simulink library "foc_blocks"  (R2020b)
settings: Solver=ode45  StartTime=0.0  StopTime=10.0  RelTol=1e-3  EnableMultiTasking=on
values from neighbouring files (symbols this model uses):
  ClockFrequency = 100    [setup_DF_fixp16_alu_av.m]    (also in setup_sim_DF_fixp16_alu.m; setup_verify_DF_fixp16_alu.m)
  constfractionlengthIn = 10    [setup_DF_fixp16_alu_av.m]    (also in setup_sim_DF_fixp16_alu.m; setup_verify_DF_fixp16_alu.m)
  constwordlengthIn = 16    [setup_DF_fixp16_alu_av.m]    (also in setup_sim_DF_fixp16_alu.m; setup_verify_DF_fixp16_alu.m)
  DSPBASampleTime = FoldingFactor / (ClockFrequency * 1e6)    (= 5e-06)    [setup_DF_fixp16_alu_av.m]    (also in setup_sim_DF_fixp16_alu.m; setup_verify_DF_fixp16_alu.m)
  FoldingFactor = 500    [setup_DF_fixp16_alu_av.m]    (also in setup_sim_DF_fixp16_alu.m; setup_verify_DF_fixp16_alu.m)
undefined symbols (not defined in the file or in its folder): AdvDSPBChannelOutDisplay, dpoly, dspba_ChannelInVis, dspba_ChannelOutVis, dspba_internal_get_channel_ports, evalAionMaskParam, latency, primtype, value, x
libraries: DSPBAPrim x559, AlteraGenericMotorLibrary x20, $bdroot x9, DSPBAUtilities x4, DSPBAControl x4
(part 3 of 6)

== system foc_blocks/FL_fixp16/SVM ==
  tmax : Inport
  ABin : Inport  Port=2
  Convert1 : DSPBAPrim/Convert  primtype=convert  nInputs=1  nOutputs=1  omode=Specify via dialog  otype=sfix(32)  scale=2^-0  rndmethod=Biased  factor=1  satmethod=None  shift_vec=[0 1 2 -1]  value=round([0:255]/17)  inPortNames=[' '; ' ';]  outPortNames=[' '; 'c']  dspbaimage=dspba_prim.jpg  text=fprintf('convert');  style=Optimised  visibilities=8+64+256+2^17  clipdetect=off  floatPrecision=float32_m23  advOptions=[]  version=20130211
  Demux : Demux  Outputs=2
  Mod : Subsystem
  Mult : DSPBAPrim/Mult  primtype=mult  nInputs=2  nOutputs=1  omode=Inherit via internal rule  otype=constOTypeMult  scale=constScaleIn  rndmethod=Unbiased  factor=1  satmethod=Symmetric  shift_vec=[0 1 2 -1]  value=0  inPortNames=[' '; ' ';]  outPortNames=[' ']  dspbaimage=dspba_prim.jpg  text=fprintf('X');  style=Optimised  visibilities=8  floatPrecision=float32_m23  floatRounding=correct  advOptions=[]  version=20130115
  Mux : Mux  Inputs=3
  ReinterpretCast1 : DSPBAPrim/ReinterpretCast  primtype=reinterpret  nInputs=1  nOutputs=1  omode=Specify via dialog  otype=sfix(33)  scale=2^-15  rndmethod=Unbiased  factor=1  satmethod=Symmetric  shift_vec=[0 1 2 -1]  value=0  inPortNames=[' '; ' ';]  outPortNames=[' ']  dspbaimage=dspba_prim.jpg  text=fprintf('Reinterp\nCast', value);  style=Optimised  visibilities=8  floatPrecision=float32_m23  version=20120601
  SectorSel : Subsystem
  rotv : Subsystem
  Out_uvw : Outport
  Out_sect : Outport  Port=2
  wires:
  Convert1/1 -> Demux/1
  ReinterpretCast1/1 -> Convert1/1
  Mult/1 -> ReinterpretCast1/1
  Mod/3(Out_w) -> Mux/3
  Mod/2(Out_v) -> Mux/2
  tmax/1 -> Mod/5(Max), Mult/2
  Mod/1(Out_u) -> Mux/1
  rotv/5(D3BA) -> Mod/8(B3m)
  rotv/6(S3BAm) -> Mod/7(B3p)
  rotv/4(uA) -> Mod/6(A)
  Demux/2 -> rotv/2(Bin), SectorSel/2(B)
  rotv/1(S) -> SectorSel/3(Sum), Mod/4(Sum)
  rotv/3(uB) -> Mod/2(B)
  rotv/2(DBA) -> SectorSel/1(D), Mod/1(D)
  Demux/1 -> rotv/1(Ain)
  ABin/1 -> Mult/1
  Mux/1 -> Out_uvw/1
  SectorSel/1(sel) -> Mod/3(Sel), Out_sect/1

== system foc_blocks/FL_fixp16_filt/FP_CP1_DSPBA ==
  note: Park & Clarke Transform
  note: Feedback Current
  note: Sin/Cos Electrical Angle
  I_uw : Inport
  cos_phi_el : Inport  Port=2
  sin_phi_el : Inport  Port=3
  Add : DSPBAPrim/Add  primtype=add  nInputs=evalAionMaskParam(gcb,'value',1)  nOutputs=1  omode=Inherit via internal rule  otype=sfix(16)  scale=2^-15  rndmethod=Unbiased  factor=1  satmethod=Symmetric  shift_vec=[0 1 2 -1]  value=2  inPortNames=[' '; ' ';]  outPortNames=[' ']  dspbaimage=dspba_prim.jpg  text=fprintf('+');  style=Optimised  visibilities=1032  genFPC=off  floatRounding=correct  advOptions=[]  version=20130821
  Add1 : DSPBAPrim/Add  primtype=add  nInputs=evalAionMaskParam(gcb,'value',1)  nOutputs=1  omode=Inherit via internal rule  otype=sfix(16)  scale=2^-15  rndmethod=Unbiased  factor=1  satmethod=Symmetric  shift_vec=[0 1 2 -1]  value=2  inPortNames=[' '; ' ';]  outPortNames=[' ']  dspbaimage=dspba_prim.jpg  text=fprintf('+');  style=Optimised  visibilities=1032  genFPC=off  floatRounding=correct  advOptions=[]  version=20130821
  Altera DSP Builder Advanced : AlteraGenericMotorLibrary/FP_Cur_Ctrl_DSPBA/Altera DSP Builder Advanced  SystemSampleTime=-1  VariantActivationTime=update diagram  Latency=0  AutoFrameSizeCalculation=off
  Demux1 : Demux  Outputs=2
  FixedGain : Subsystem  mask{constVal=2}
      mask prompts: constVal "Gain"
      mask Display: color('w');fprintf('Fixed Gain\n%s', num2str(constVal));port_label('input',1,'a');port_label('output',1,'q');
  FixedGain1 : Subsystem  mask{constVal=-1/sqrt(3)}
      mask prompts: constVal "Gain"
      mask Display: color('w');fprintf('Fixed Gain\n%s', num2str(constVal));port_label('input',1,'a');port_label('output',1,'q');
  Mult{,1..3} (4 alike) : DSPBAPrim/Mult  primtype=mult  nInputs=2  nOutputs=1  omode=Specify via dialog  otype=constOTypeIn  scale=constScaleIn  rndmethod=Unbiased  factor=1  satmethod=Symmetric  shift_vec=[0 1 2 -1]  value=0  inPortNames=[' '; ' ';]  outPortNames=[' ']  dspbaimage=dspba_prim.jpg  text=fprintf('X');  style=Optimised  visibilities=8  floatPrecision=float32_m23  floatRounding=correct  advOptions=[]  version=20130115
  Mux1 : Mux  Inputs=2
  Sub1 : DSPBAPrim/Sub  primtype=sub  nInputs=2  nOutputs=1  omode=Inherit via internal rule  otype=sfix(16)  scale=2^-15  rndmethod=Unbiased  factor=1  satmethod=Symmetric  shift_vec=[0 1 2 -1]  value=0  inPortNames=['+'; '-';]  outPortNames=[' ']  dspbaimage=dspba_prim.jpg  text=fprintf('-');  style=Optimised  visibilities=8  floatRounding=correct  advOptions=[]  version=20130115
  I_dq : Outport
  wires:
  Sub1/1 -> Mux1/2
  Add/1 -> Mux1/1
  Mux1/1 -> I_dq/1
  Mult3/1 -> Sub1/1
  Mult2/1 -> Sub1/2
  Mult1/1 -> Add/2
  Mult/1 -> Add/1
  cos_phi_el/1 -> Mult/2, Mult3/2
  FixedGain1/1(Out1) -> Mult1/1, Mult3/1
  Demux1/1 -> Mult/1, Mult2/2, Add1/1
  Demux1/2 -> FixedGain/1(In1)
  I_uw/1 -> Demux1/1
  sin_phi_el/1 -> Mult1/2, Mult2/1
  Add1/1 -> FixedGain1/1(In1)
  FixedGain/1(Out1) -> Add1/2

== system foc_blocks/FL_fixp16_filt/FP_Inv_Park ==
  note: Inverse Park Transform
  note: Sin/Cos Electrical Angle
  note: Direct/Quadrature Voltage
  note: Alpha/Beta Voltage
  V_dq : Inport
  cos_phi_el : Inport  Port=2
  sin_phi_el : Inport  Port=3
  Add : DSPBAPrim/Add  primtype=add  nInputs=evalAionMaskParam(gcb,'value',1)  nOutputs=1  omode=Inherit via internal rule with word growth  otype=sfix(16)  scale=2^-15  rndmethod=Unbiased  factor=1  satmethod=Symmetric  shift_vec=[0 1 2 -1]  value=2  inPortNames=[' '; ' ';]  outPortNames=[' ']  dspbaimage=dspba_prim.jpg  text=fprintf('+');  style=Optimised  visibilities=1032  genFPC=off  floatRounding=correct  advOptions=[]  version=20130821
  Altera DSP Builder Advanced : AlteraGenericMotorLibrary/FP_Cur_Ctrl_DSPBA/Altera DSP Builder Advanced  SystemSampleTime=-1  VariantActivationTime=update diagram  Latency=0  AutoFrameSizeCalculation=off
  Demux1 : Demux  Outputs=2
  Mult{,1..3} (4 alike) : DSPBAPrim/Mult  primtype=mult  nInputs=2  nOutputs=1  omode=Specify via dialog  otype=constOTypeMult  scale=constScaleIn  rndmethod=Unbiased  factor=1  satmethod=Symmetric  shift_vec=[0 1 2 -1]  value=0  inPortNames=[' '; ' ';]  outPortNames=[' ']  dspbaimage=dspba_prim.jpg  text=fprintf('X');  style=Optimised  visibilities=8  floatPrecision=float32_m23  floatRounding=correct  advOptions=[]  version=20130115
  Mux2 : Mux  Inputs=2
  Sub1 : DSPBAPrim/Sub  primtype=sub  nInputs=2  nOutputs=1  omode=Inherit via internal rule with word growth  otype=sfix(16)  scale=2^-15  rndmethod=Unbiased  factor=1  satmethod=Symmetric  shift_vec=[0 1 2 -1]  value=0  inPortNames=['+'; '-';]  outPortNames=[' ']  dspbaimage=dspba_prim.jpg  text=fprintf('-');  style=Optimised  visibilities=8  floatRounding=correct  advOptions=[]  version=20130115
  V_alpha_beta : Outport
  wires:
  Mult2/1 -> Add/1
  Mult3/1 -> Add/2
  Mult/1 -> Sub1/1
  Mult1/1 -> Sub1/2
  Demux1/1 -> Mult/1, Mult2/1  "I_d"
  cos_phi_el/1 -> Mult/2, Mult3/2
  Demux1/2 -> Mult1/1, Mult3/1  "I_q"
  sin_phi_el/1 -> Mult1/2, Mult2/2
  V_dq/1 -> Demux1/1
  Mux2/1 -> V_alpha_beta/1
  Sub1/1 -> Mux2/1
  Add/1 -> Mux2/2

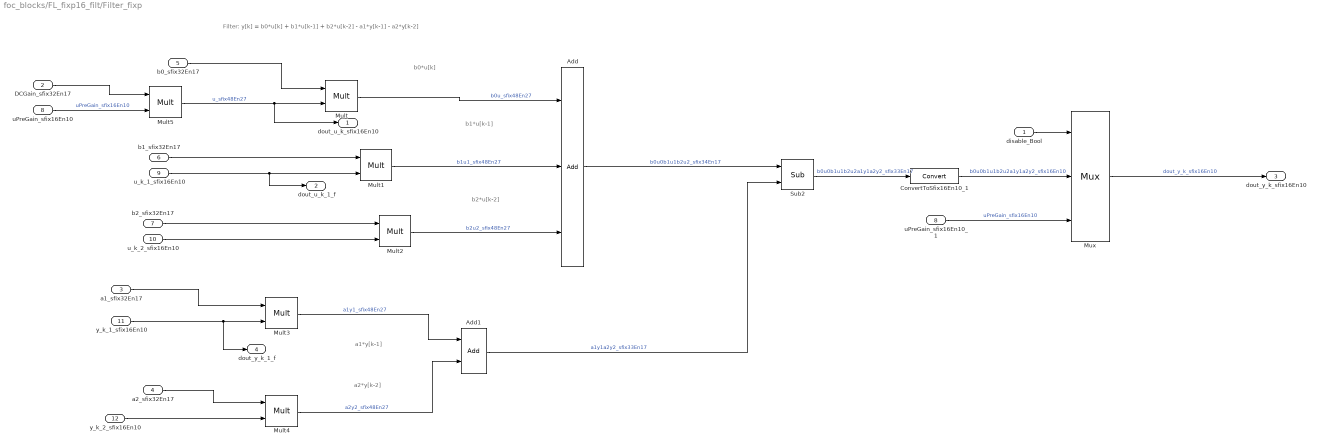
== system foc_blocks/FL_fixp16_filt/Filter_fixp ==
  note: b0*u[k]
  note: b1*u[k-1]
  note: b2*u[k-2]
  note: a1*y[k-1]
  note: a2*y[k-2]
  note: Filter: y[k] = b0*u[k] + b1*u[k-1] + b2*u[k-2] - a1*y[k-1] - a2*y[k-2]
  disable_Bool : Inport
  DCGain_sfix32En17 : Inport  Port=2
  a1_sfix32En17 : Inport  Port=3
  a2_sfix32En17 : Inport  Port=4
  b0_sfix32En17 : Inport  Port=5
  b1_sfix32En17 : Inport  Port=6
  b2_sfix32En17 : Inport  Port=7
  uPreGain_sfix16En10 : Inport  Port=8
  u_k_1_sfix16En10 : Inport  Port=9
  u_k_2_sfix16En10 : Inport  Port=10
  y_k_1_sfix16En10 : Inport  Port=11
  y_k_2_sfix16En10 : Inport  Port=12
  Add : DSPBAPrim/Add  primtype=add  nInputs=evalAionMaskParam(gcb,'value',1)  nOutputs=1  omode=Inherit via internal rule  otype=sfix(16)  scale=2^-15  rndmethod=Unbiased  factor=1  satmethod=Symmetric  shift_vec=[0 1 2 -1]  value=3  inPortNames=[' '; ' ';]  outPortNames=[' ']  dspbaimage=dspba_prim.jpg  text=fprintf('+');  style=Optimised  visibilities=1032  genFPC=off  floatRounding=correct  advOptions=[]  version=20130821
  Add1 : DSPBAPrim/Add  primtype=add  nInputs=evalAionMaskParam(gcb,'value',1)  nOutputs=1  omode=Inherit via internal rule  otype=sfix(16)  scale=2^-15  rndmethod=Unbiased  factor=1  satmethod=Symmetric  shift_vec=[0 1 2 -1]  value=2  inPortNames=[' '; ' ';]  outPortNames=[' ']  dspbaimage=dspba_prim.jpg  text=fprintf('+');  style=Optimised  visibilities=1032  genFPC=off  floatRounding=correct  advOptions=[]  version=20130821
  ConvertToSfix16En10_1 : DSPBAPrim/Convert  primtype=convert  nInputs=1  nOutputs=1  omode=Specify via dialog  otype=constOTypeIn  scale=constScaleIn  rndmethod=Truncate  factor=1  satmethod=None  shift_vec=[0 1 2 -1]  value=round([0:255]/17)  inPortNames=[' '; ' ';]  outPortNames=[' '; 'c']  dspbaimage=dspba_prim.jpg  text=fprintf('convert');  style=Optimised  visibilities=8+64+256+2^17  clipdetect=off  floatPrecision=float32_m23  advOptions=[]  version=20130211
  Mult{,1..4} (5 alike) : DSPBAPrim/Mult  primtype=mult  nInputs=2  nOutputs=1  omode=Specify via dialog  otype=constOTypeFilterCoeffs  scale=constScaleFilterCoeffs  rndmethod=Unbiased  factor=1  satmethod=Symmetric  shift_vec=[0 1 2 -1]  value=0  inPortNames=[' '; ' ';]  outPortNames=[' ']  dspbaimage=dspba_prim.jpg  text=fprintf('X');  style=Optimised  visibilities=8  floatPrecision=float32_m23  floatRounding=correct  advOptions=[]  version=20130115
  Mult5 : DSPBAPrim/Mult  primtype=mult  nInputs=2  nOutputs=1  omode=Specify via dialog  otype=constOTypeIn  scale=constScaleIn  rndmethod=Unbiased  factor=1  satmethod=Symmetric  shift_vec=[0 1 2 -1]  value=0  inPortNames=[' '; ' ';]  outPortNames=[' ']  dspbaimage=dspba_prim.jpg  text=fprintf('X');  style=Optimised  visibilities=8  floatPrecision=float32_m23  floatRounding=correct  advOptions=[]  version=20130115
  Mux : DSPBAPrim/Mux  primtype=mux  nInputs=evalAionMaskParam(gcb,'value',1)+1  nOutputs=1  omode=Inherit via internal rule  otype=constOTypeFromFOC  scale=constScaleFromFOC  rndmethod=Unbiased  factor=1  satmethod=Symmetric  shift_vec=[0 1 2 -1]  value=2  inPortNames=['s'; 'd0'; 'd1'; 'd2'; 'd3'; 'd4'; 'd5'; 'd6'; 'd7'; 'd8'; 'd9';]  outPortNames=[' ']  dspbaimage=dspba_prim.jpg  text=fprintf('%s', primtype);  style=Optimised  visibilities=1032  version=20131025
  Sub2 : DSPBAPrim/Sub  primtype=sub  nInputs=2  nOutputs=1  omode=Inherit via internal rule  otype=sfix(16)  scale=2^-15  rndmethod=Unbiased  factor=1  satmethod=Symmetric  shift_vec=[0 1 2 -1]  value=0  inPortNames=['+'; '-';]  outPortNames=[' ']  dspbaimage=dspba_prim.jpg  text=fprintf('-');  style=Optimised  visibilities=8  floatRounding=correct  advOptions=[]  version=20130115
  uPreGain_sfix16En10_1 : InportShadow  Port=8
  dout_u_k_sfix16En10 : Outport
  dout_u_k_1_f : Outport  Port=2
  dout_y_k_sfix16En10 : Outport  Port=3
  dout_y_k_1_f : Outport  Port=4
  wires:
  Mult4/1 -> Add1/2  "a2y2_sfix48En27"
  Mult3/1 -> Add1/1  "a1y1_sfix48En27"
  Add1/1 -> Sub2/2  "a1y1a2y2_sfix33En17"
  Add/1 -> Sub2/1  "b0u0b1u1b2u2_sfix34En17"
  Mult1/1 -> Add/2  "b1u1_sfix48En27"
  Mult/1 -> Add/1  "b0u_sfix48En27"
  Mult2/1 -> Add/3  "b2u2_sfix48En27"
  Mult5/1 -> dout_u_k_sfix16En10/1, Mult/2  "u_sfix48En27"
  disable_Bool/1 -> Mux/1
  Sub2/1 -> ConvertToSfix16En10_1/1  "b0u0b1u1b2u2a1y1a2y2_sfix33En17"
  Mux/1 -> dout_y_k_sfix16En10/1  "dout_y_k_sfix16En10"
  DCGain_sfix32En17/1 -> Mult5/1
  uPreGain_sfix16En10/1 -> Mult5/2  "uPreGain_sfix16En10"
  uPreGain_sfix16En10_1/1 -> Mux/3  "uPreGain_sfix16En10"
  b0_sfix32En17/1 -> Mult/1
  b2_sfix32En17/1 -> Mult2/1
  b1_sfix32En17/1 -> Mult1/1
  a1_sfix32En17/1 -> Mult3/1
  a2_sfix32En17/1 -> Mult4/1
  ConvertToSfix16En10_1/1 -> Mux/2  "b0u0b1u1b2u2a1y1a2y2_sfix16En10"
  u_k_1_sfix16En10/1 -> dout_u_k_1_f/1, Mult1/2
  u_k_2_sfix16En10/1 -> Mult2/2
  y_k_1_sfix16En10/1 -> dout_y_k_1_f/1, Mult3/2
  y_k_2_sfix16En10/1 -> Mult4/2

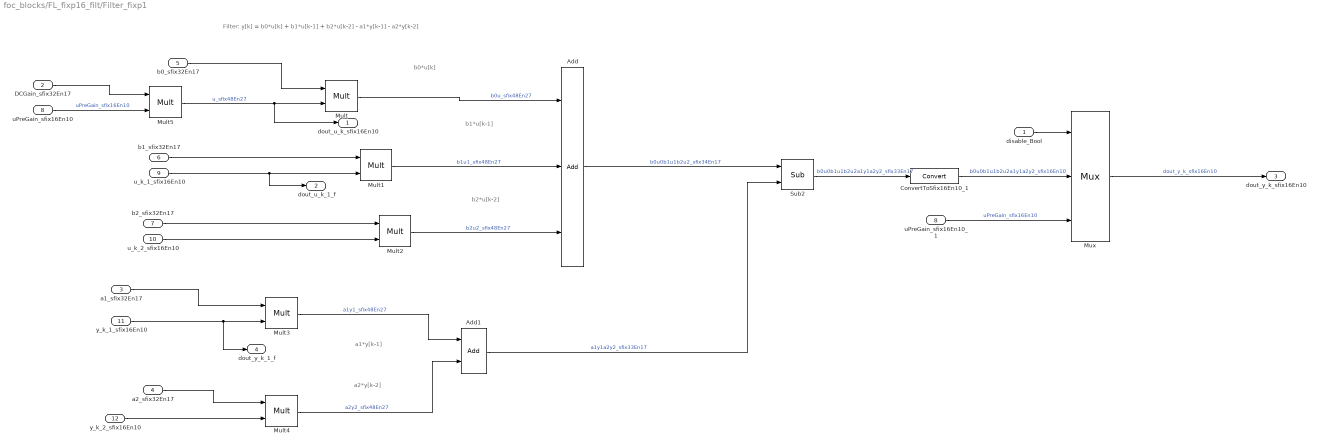
== system foc_blocks/FL_fixp16_filt/Filter_fixp1 ==
  note: b0*u[k]
  note: b1*u[k-1]
  note: b2*u[k-2]
  note: a1*y[k-1]
  note: a2*y[k-2]
  note: Filter: y[k] = b0*u[k] + b1*u[k-1] + b2*u[k-2] - a1*y[k-1] - a2*y[k-2]
  disable_Bool : Inport
  DCGain_sfix32En17 : Inport  Port=2
  a1_sfix32En17 : Inport  Port=3
  a2_sfix32En17 : Inport  Port=4
  b0_sfix32En17 : Inport  Port=5
  b1_sfix32En17 : Inport  Port=6
  b2_sfix32En17 : Inport  Port=7
  uPreGain_sfix16En10 : Inport  Port=8
  u_k_1_sfix16En10 : Inport  Port=9
  u_k_2_sfix16En10 : Inport  Port=10
  y_k_1_sfix16En10 : Inport  Port=11
  y_k_2_sfix16En10 : Inport  Port=12
  Add : DSPBAPrim/Add  primtype=add  nInputs=evalAionMaskParam(gcb,'value',1)  nOutputs=1  omode=Inherit via internal rule  otype=sfix(16)  scale=2^-15  rndmethod=Unbiased  factor=1  satmethod=Symmetric  shift_vec=[0 1 2 -1]  value=3  inPortNames=[' '; ' ';]  outPortNames=[' ']  dspbaimage=dspba_prim.jpg  text=fprintf('+');  style=Optimised  visibilities=1032  genFPC=off  floatRounding=correct  advOptions=[]  version=20130821
  Add1 : DSPBAPrim/Add  primtype=add  nInputs=evalAionMaskParam(gcb,'value',1)  nOutputs=1  omode=Inherit via internal rule  otype=sfix(16)  scale=2^-15  rndmethod=Unbiased  factor=1  satmethod=Symmetric  shift_vec=[0 1 2 -1]  value=2  inPortNames=[' '; ' ';]  outPortNames=[' ']  dspbaimage=dspba_prim.jpg  text=fprintf('+');  style=Optimised  visibilities=1032  genFPC=off  floatRounding=correct  advOptions=[]  version=20130821
  ConvertToSfix16En10_1 : DSPBAPrim/Convert  primtype=convert  nInputs=1  nOutputs=1  omode=Specify via dialog  otype=constOTypeIn  scale=constScaleIn  rndmethod=Truncate  factor=1  satmethod=None  shift_vec=[0 1 2 -1]  value=round([0:255]/17)  inPortNames=[' '; ' ';]  outPortNames=[' '; 'c']  dspbaimage=dspba_prim.jpg  text=fprintf('convert');  style=Optimised  visibilities=8+64+256+2^17  clipdetect=off  floatPrecision=float32_m23  advOptions=[]  version=20130211
  Mult{,1..4} (5 alike) : DSPBAPrim/Mult  primtype=mult  nInputs=2  nOutputs=1  omode=Specify via dialog  otype=constOTypeFilterCoeffs  scale=constScaleFilterCoeffs  rndmethod=Unbiased  factor=1  satmethod=Symmetric  shift_vec=[0 1 2 -1]  value=0  inPortNames=[' '; ' ';]  outPortNames=[' ']  dspbaimage=dspba_prim.jpg  text=fprintf('X');  style=Optimised  visibilities=8  floatPrecision=float32_m23  floatRounding=correct  advOptions=[]  version=20130115
  Mult5 : DSPBAPrim/Mult  primtype=mult  nInputs=2  nOutputs=1  omode=Specify via dialog  otype=constOTypeIn  scale=constScaleIn  rndmethod=Unbiased  factor=1  satmethod=Symmetric  shift_vec=[0 1 2 -1]  value=0  inPortNames=[' '; ' ';]  outPortNames=[' ']  dspbaimage=dspba_prim.jpg  text=fprintf('X');  style=Optimised  visibilities=8  floatPrecision=float32_m23  floatRounding=correct  advOptions=[]  version=20130115
  Mux : DSPBAPrim/Mux  primtype=mux  nInputs=evalAionMaskParam(gcb,'value',1)+1  nOutputs=1  omode=Inherit via internal rule  otype=constOTypeFromFOC  scale=constScaleFromFOC  rndmethod=Unbiased  factor=1  satmethod=Symmetric  shift_vec=[0 1 2 -1]  value=2  inPortNames=['s'; 'd0'; 'd1'; 'd2'; 'd3'; 'd4'; 'd5'; 'd6'; 'd7'; 'd8'; 'd9';]  outPortNames=[' ']  dspbaimage=dspba_prim.jpg  text=fprintf('%s', primtype);  style=Optimised  visibilities=1032  version=20131025
  Sub2 : DSPBAPrim/Sub  primtype=sub  nInputs=2  nOutputs=1  omode=Inherit via internal rule  otype=sfix(16)  scale=2^-15  rndmethod=Unbiased  factor=1  satmethod=Symmetric  shift_vec=[0 1 2 -1]  value=0  inPortNames=['+'; '-';]  outPortNames=[' ']  dspbaimage=dspba_prim.jpg  text=fprintf('-');  style=Optimised  visibilities=8  floatRounding=correct  advOptions=[]  version=20130115
  uPreGain_sfix16En10_1 : InportShadow  Port=8
  dout_u_k_sfix16En10 : Outport
  dout_u_k_1_f : Outport  Port=2
  dout_y_k_sfix16En10 : Outport  Port=3
  dout_y_k_1_f : Outport  Port=4
  wires:
  Mult4/1 -> Add1/2  "a2y2_sfix48En27"
  Mult3/1 -> Add1/1  "a1y1_sfix48En27"
  Add1/1 -> Sub2/2  "a1y1a2y2_sfix33En17"
  Add/1 -> Sub2/1  "b0u0b1u1b2u2_sfix34En17"
  Mult1/1 -> Add/2  "b1u1_sfix48En27"
  Mult/1 -> Add/1  "b0u_sfix48En27"
  Mult2/1 -> Add/3  "b2u2_sfix48En27"
  Mult5/1 -> dout_u_k_sfix16En10/1, Mult/2  "u_sfix48En27"
  disable_Bool/1 -> Mux/1
  Sub2/1 -> ConvertToSfix16En10_1/1  "b0u0b1u1b2u2a1y1a2y2_sfix33En17"
  Mux/1 -> dout_y_k_sfix16En10/1  "dout_y_k_sfix16En10"
  DCGain_sfix32En17/1 -> Mult5/1
  uPreGain_sfix16En10/1 -> Mult5/2  "uPreGain_sfix16En10"
  uPreGain_sfix16En10_1/1 -> Mux/3  "uPreGain_sfix16En10"
  b0_sfix32En17/1 -> Mult/1
  b2_sfix32En17/1 -> Mult2/1
  b1_sfix32En17/1 -> Mult1/1
  a1_sfix32En17/1 -> Mult3/1
  a2_sfix32En17/1 -> Mult4/1
  ConvertToSfix16En10_1/1 -> Mux/2  "b0u0b1u1b2u2a1y1a2y2_sfix16En10"
  u_k_1_sfix16En10/1 -> dout_u_k_1_f/1, Mult1/2
  u_k_2_sfix16En10/1 -> Mult2/2
  y_k_1_sfix16En10/1 -> dout_y_k_1_f/1, Mult3/2
  y_k_2_sfix16En10/1 -> Mult4/2

== system foc_blocks/FL_fixp16_filt/Fixed Saturate1 ==
  In1 : Inport
  limit : Inport  Port=2
  MinMax : DSPBAPrim/MinMax  primtype=minmaxfunc  nInputs=2  nOutputs=1  omode=Specify via dialog  otype=constOTypeIn  scale=constScaleIn  rndmethod=Unbiased  factor=1  satmethod=Symmetric  shift_vec=[0 1 2 -1]  value=0  inPortNames=[' '; ' ';]  outPortNames=[' ']  dspbaimage=dspba_prim.jpg  text=disp('min');  style=Optimised  visibilities=8+2^17  functionExpr=min  advOptions=[]  version=20121130
  MinMax1 : DSPBAPrim/MinMax  primtype=minmaxfunc  nInputs=2  nOutputs=1  omode=Specify via dialog  otype=constOTypeIn  scale=constScaleIn  rndmethod=Unbiased  factor=1  satmethod=Symmetric  shift_vec=[0 1 2 -1]  value=0  inPortNames=[' '; ' ';]  outPortNames=[' ']  dspbaimage=dspba_prim.jpg  text=disp('min');  style=Optimised  visibilities=8+2^17  functionExpr=max  advOptions=[]  version=20121130
  Sub : DSPBAPrim/Sub  primtype=sub  nInputs=2  nOutputs=1  omode=Inherit via internal rule  otype=sfix(16)  scale=2^-15  rndmethod=Unbiased  factor=1  satmethod=Symmetric  shift_vec=[0 1 2 -1]  value=0  inPortNames=['+'; '-';]  outPortNames=[' ']  dspbaimage=dspba_prim.jpg  text=fprintf('-');  style=Optimised  visibilities=8  floatRounding=correct  advOptions=[]  version=20130115
  const1 : DSPBAPrim/Const  primtype=const  nInputs=0  nOutputs=1  omode=Specify via dialog  otype=constOTypeIn  scale=constScaleIn  rndmethod=Unbiased  factor=1  satmethod=Symmetric  shift_vec=[0 1 2 -1]  value=0  inPortNames=['+'; '+';]  outPortNames=[' ']  dspbaimage=dspba_prim.jpg  text=fprintf('%s', num2str(value));  style=Optimised  visibilities=8 + 1024  floatPrecision=float32_m23  version=20120820
  Out1 : Outport
  wires:
  limit/1 -> MinMax/1, Sub/2
  const1/1 -> Sub/1
  In1/1 -> MinMax/2
  Sub/1 -> MinMax1/2
  MinMax1/1 -> Out1/1
  MinMax/1 -> MinMax1/1

== system foc_blocks/FL_fixp16_filt/Fixed Saturate2 ==
  In1 : Inport
  limit : Inport  Port=2
  MinMax : DSPBAPrim/MinMax  primtype=minmaxfunc  nInputs=2  nOutputs=1  omode=Specify via dialog  otype=constOTypeIn  scale=constScaleIn  rndmethod=Unbiased  factor=1  satmethod=Symmetric  shift_vec=[0 1 2 -1]  value=0  inPortNames=[' '; ' ';]  outPortNames=[' ']  dspbaimage=dspba_prim.jpg  text=disp('min');  style=Optimised  visibilities=8+2^17  functionExpr=min  advOptions=[]  version=20121130
  MinMax1 : DSPBAPrim/MinMax  primtype=minmaxfunc  nInputs=2  nOutputs=1  omode=Specify via dialog  otype=constOTypeIn  scale=constScaleIn  rndmethod=Unbiased  factor=1  satmethod=Symmetric  shift_vec=[0 1 2 -1]  value=0  inPortNames=[' '; ' ';]  outPortNames=[' ']  dspbaimage=dspba_prim.jpg  text=disp('min');  style=Optimised  visibilities=8+2^17  functionExpr=max  advOptions=[]  version=20121130
  Sub : DSPBAPrim/Sub  primtype=sub  nInputs=2  nOutputs=1  omode=Inherit via internal rule  otype=sfix(16)  scale=2^-15  rndmethod=Unbiased  factor=1  satmethod=Symmetric  shift_vec=[0 1 2 -1]  value=0  inPortNames=['+'; '-';]  outPortNames=[' ']  dspbaimage=dspba_prim.jpg  text=fprintf('-');  style=Optimised  visibilities=8  floatRounding=correct  advOptions=[]  version=20130115
  const1 : DSPBAPrim/Const  primtype=const  nInputs=0  nOutputs=1  omode=Specify via dialog  otype=constOTypeIn  scale=constScaleIn  rndmethod=Unbiased  factor=1  satmethod=Symmetric  shift_vec=[0 1 2 -1]  value=0  inPortNames=['+'; '+';]  outPortNames=[' ']  dspbaimage=dspba_prim.jpg  text=fprintf('%s', num2str(value));  style=Optimised  visibilities=8 + 1024  floatPrecision=float32_m23  version=20120820
  Out1 : Outport
  wires:
  MinMax/1 -> MinMax1/1
  MinMax1/1 -> Out1/1
  Sub/1 -> MinMax1/2
  In1/1 -> MinMax/2
  const1/1 -> Sub/1
  limit/1 -> Sub/2, MinMax/1

== system foc_blocks/FL_fixp16_filt/PI_Ctrl_D_DSPBA ==
  note: Simple Proportional + Integral (PI) Controller
  note: Error Input
  note: Proportional Gain
  note: Integral Gain
  note: Saturate
  note: Saturate
  note: Correction Output
  note: Integral Input
  note: Integral Output
  note: Kp
  note: Ki
  note: Saturation limit
  PI_in : Inport
  Integral_in : Inport  Port=2
  Kp_in : Inport  Port=3
  Ki_in : Inport  Port=4
  Add1 : DSPBAPrim/Add  primtype=add  nInputs=evalAionMaskParam(gcb,'value',1)  nOutputs=1  omode=Inherit via internal rule with word growth  otype=sfix(16)  scale=2^-15  rndmethod=Unbiased  factor=1  satmethod=Symmetric  shift_vec=[0 1 2 -1]  value=2  inPortNames=[' '; ' ';]  outPortNames=[' ']  dspbaimage=dspba_prim.jpg  text=fprintf('+');  style=Optimised  visibilities=1032  genFPC=off  floatRounding=correct  advOptions=[]  version=20130821
  Add4 : DSPBAPrim/Add  primtype=add  nInputs=evalAionMaskParam(gcb,'value',1)  nOutputs=1  omode=Inherit via internal rule with word growth  otype=sfix(16)  scale=2^-15  rndmethod=Unbiased  factor=1  satmethod=Symmetric  shift_vec=[0 1 2 -1]  value=2  inPortNames=[' '; ' ';]  outPortNames=[' ']  dspbaimage=dspba_prim.jpg  text=fprintf('+');  style=Optimised  visibilities=1032  genFPC=off  floatRounding=correct  advOptions=[]  version=20130821
  Altera DSP Builder Advanced : AlteraGenericMotorLibrary/FP_Cur_Ctrl_DSPBA/Altera DSP Builder Advanced  SystemSampleTime=-1  VariantActivationTime=update diagram  Latency=0  AutoFrameSizeCalculation=off
  Fixed Saturate1 : Subsystem
  Fixed Saturate2 : Subsystem
  Limit : DSPBAPrim/Const  primtype=const  nInputs=0  nOutputs=1  omode=Specify via dialog  otype=constOTypeIn  scale=constScaleIn  rndmethod=Unbiased  factor=1  satmethod=Symmetric  shift_vec=[0 1 2 -1]  value=0.95*2^(constwordlengthIn-constfractionlengthIn-1)  inPortNames=['+'; '+';]  outPortNames=[' ']  dspbaimage=dspba_prim.jpg  text=fprintf('%s', num2str(value));  style=Optimised  visibilities=8 + 1024  floatPrecision=float32_m23  version=20120820
  Mult : DSPBAPrim/Mult  primtype=mult  nInputs=2  nOutputs=1  omode=Specify via dialog  otype=constOTypeMult  scale=constScaleIn  rndmethod=Unbiased  factor=1  satmethod=Symmetric  shift_vec=[0 1 2 -1]  value=0  inPortNames=[' '; ' ';]  outPortNames=[' ']  dspbaimage=dspba_prim.jpg  text=fprintf('X');  style=Optimised  visibilities=8  floatPrecision=float32_m23  floatRounding=correct  advOptions=[]  version=20130115
  Mult1 : DSPBAPrim/Mult  primtype=mult  nInputs=2  nOutputs=1  omode=Specify via dialog  otype=constOTypeMult  scale=constScaleIn  rndmethod=Unbiased  factor=1  satmethod=Symmetric  shift_vec=[0 1 2 -1]  value=0  inPortNames=[' '; ' ';]  outPortNames=[' ']  dspbaimage=dspba_prim.jpg  text=fprintf('X');  style=Optimised  visibilities=8  floatPrecision=float32_m23  floatRounding=correct  advOptions=[]  version=20130115
  PI_out : Outport
  I_out : Outport  Port=2
  wires:
  Fixed Saturate1/1(Out1) -> PI_out/1
  Add1/1 -> Fixed Saturate1/1(In1)
  PI_in/1 -> Mult1/1, Mult/1
  Mult/1 -> Add1/1
  Fixed Saturate2/1(Out1) -> Add1/2, I_out/1
  Mult1/1 -> Add4/1
  Add4/1 -> Fixed Saturate2/1(In1)
  Integral_in/1 -> Add4/2
  Kp_in/1 -> Mult/2
  Ki_in/1 -> Mult1/2
  Limit/1 -> Fixed Saturate2/2(limit), Fixed Saturate1/2(limit)

== system foc_blocks/FL_fixp16_filt/PI_Ctrl_D_DSPBA1 ==
  note: Ki
  note: Kp
  note: Integral Output
  note: Integral Input
  note: Correction Output
  note: Saturate
  note: Saturate
  note: Integral Gain
  note: Proportional Gain
  note: Error Input
  note: Simple Proportional + Integral (PI) Controller
  note: Saturation limit
  PI_in : Inport
  Integral_in : Inport  Port=2
  Kp_in : Inport  Port=3
  Ki_in : Inport  Port=4
  Add1 : DSPBAPrim/Add  primtype=add  nInputs=evalAionMaskParam(gcb,'value',1)  nOutputs=1  omode=Inherit via internal rule with word growth  otype=sfix(16)  scale=2^-15  rndmethod=Unbiased  factor=1  satmethod=Symmetric  shift_vec=[0 1 2 -1]  value=2  inPortNames=[' '; ' ';]  outPortNames=[' ']  dspbaimage=dspba_prim.jpg  text=fprintf('+');  style=Optimised  visibilities=1032  genFPC=off  floatRounding=correct  advOptions=[]  version=20130821
  Add4 : DSPBAPrim/Add  primtype=add  nInputs=evalAionMaskParam(gcb,'value',1)  nOutputs=1  omode=Inherit via internal rule with word growth  otype=sfix(16)  scale=2^-15  rndmethod=Unbiased  factor=1  satmethod=Symmetric  shift_vec=[0 1 2 -1]  value=2  inPortNames=[' '; ' ';]  outPortNames=[' ']  dspbaimage=dspba_prim.jpg  text=fprintf('+');  style=Optimised  visibilities=1032  genFPC=off  floatRounding=correct  advOptions=[]  version=20130821
  Altera DSP Builder Advanced : AlteraGenericMotorLibrary/FP_Cur_Ctrl_DSPBA/Altera DSP Builder Advanced  SystemSampleTime=-1  VariantActivationTime=update diagram  Latency=0  AutoFrameSizeCalculation=off
  Fixed Saturate1 : Subsystem
  Fixed Saturate2 : Subsystem
  Limit : DSPBAPrim/Const  primtype=const  nInputs=0  nOutputs=1  omode=Specify via dialog  otype=constOTypeIn  scale=constScaleIn  rndmethod=Unbiased  factor=1  satmethod=Symmetric  shift_vec=[0 1 2 -1]  value=0.95*2^(constwordlengthIn-constfractionlengthIn-1)  inPortNames=['+'; '+';]  outPortNames=[' ']  dspbaimage=dspba_prim.jpg  text=fprintf('%s', num2str(value));  style=Optimised  visibilities=8 + 1024  floatPrecision=float32_m23  version=20120820
  Mult : DSPBAPrim/Mult  primtype=mult  nInputs=2  nOutputs=1  omode=Specify via dialog  otype=constOTypeMult  scale=constScaleIn  rndmethod=Unbiased  factor=1  satmethod=Symmetric  shift_vec=[0 1 2 -1]  value=0  inPortNames=[' '; ' ';]  outPortNames=[' ']  dspbaimage=dspba_prim.jpg  text=fprintf('X');  style=Optimised  visibilities=8  floatPrecision=float32_m23  floatRounding=correct  advOptions=[]  version=20130115
  Mult1 : DSPBAPrim/Mult  primtype=mult  nInputs=2  nOutputs=1  omode=Specify via dialog  otype=constOTypeMult  scale=constScaleIn  rndmethod=Unbiased  factor=1  satmethod=Symmetric  shift_vec=[0 1 2 -1]  value=0  inPortNames=[' '; ' ';]  outPortNames=[' ']  dspbaimage=dspba_prim.jpg  text=fprintf('X');  style=Optimised  visibilities=8  floatPrecision=float32_m23  floatRounding=correct  advOptions=[]  version=20130115
  PI_out : Outport
  I_out : Outport  Port=2
  wires:
  Ki_in/1 -> Mult1/2
  Kp_in/1 -> Mult/2
  Integral_in/1 -> Add4/2
  Add4/1 -> Fixed Saturate2/1(In1)
  Mult1/1 -> Add4/1
  Fixed Saturate2/1(Out1) -> I_out/1, Add1/2
  Mult/1 -> Add1/1
  PI_in/1 -> Mult/1, Mult1/1
  Add1/1 -> Fixed Saturate1/1(In1)
  Fixed Saturate1/1(Out1) -> PI_out/1
  Limit/1 -> Fixed Saturate1/2(limit), Fixed Saturate2/2(limit)

== system foc_blocks/FL_fixp16_filt/SVM ==
  tmax : Inport
  ABin : Inport  Port=2
  Convert1 : DSPBAPrim/Convert  primtype=convert  nInputs=1  nOutputs=1  omode=Specify via dialog  otype=sfix(32)  scale=2^-0  rndmethod=Biased  factor=1  satmethod=None  shift_vec=[0 1 2 -1]  value=round([0:255]/17)  inPortNames=[' '; ' ';]  outPortNames=[' '; 'c']  dspbaimage=dspba_prim.jpg  text=fprintf('convert');  style=Optimised  visibilities=8+64+256+2^17  clipdetect=off  floatPrecision=float32_m23  advOptions=[]  version=20130211
  Demux : Demux  Outputs=2
  Mod : Subsystem
  Mult : DSPBAPrim/Mult  primtype=mult  nInputs=2  nOutputs=1  omode=Inherit via internal rule  otype=constOTypeMult  scale=constScaleIn  rndmethod=Unbiased  factor=1  satmethod=Symmetric  shift_vec=[0 1 2 -1]  value=0  inPortNames=[' '; ' ';]  outPortNames=[' ']  dspbaimage=dspba_prim.jpg  text=fprintf('X');  style=Optimised  visibilities=8  floatPrecision=float32_m23  floatRounding=correct  advOptions=[]  version=20130115
  Mux : Mux  Inputs=3
  ReinterpretCast1 : DSPBAPrim/ReinterpretCast  primtype=reinterpret  nInputs=1  nOutputs=1  omode=Specify via dialog  otype=sfix(33)  scale=2^-15  rndmethod=Unbiased  factor=1  satmethod=Symmetric  shift_vec=[0 1 2 -1]  value=0  inPortNames=[' '; ' ';]  outPortNames=[' ']  dspbaimage=dspba_prim.jpg  text=fprintf('Reinterp\nCast', value);  style=Optimised  visibilities=8  floatPrecision=float32_m23  version=20120601
  SectorSel : Subsystem
  rotv : Subsystem
  Out_uvw : Outport
  Out_sect : Outport  Port=2
  wires:
  SectorSel/1(sel) -> Out_sect/1, Mod/3(Sel)
  Mux/1 -> Out_uvw/1
  ABin/1 -> Mult/1
  Demux/1 -> rotv/1(Ain)
  rotv/2(DBA) -> Mod/1(D), SectorSel/1(D)
  rotv/3(uB) -> Mod/2(B)
  rotv/1(S) -> Mod/4(Sum), SectorSel/3(Sum)
  Demux/2 -> SectorSel/2(B), rotv/2(Bin)
  rotv/4(uA) -> Mod/6(A)
  rotv/6(S3BAm) -> Mod/7(B3p)
  rotv/5(D3BA) -> Mod/8(B3m)
  Mod/1(Out_u) -> Mux/1
  tmax/1 -> Mult/2, Mod/5(Max)
  Mod/2(Out_v) -> Mux/2
  Mod/3(Out_w) -> Mux/3
  Mult/1 -> ReinterpretCast1/1
  ReinterpretCast1/1 -> Convert1/1
  Convert1/1 -> Demux/1

== system foc_blocks/FL_float/FPSaturate1 ==
  a : Inport
  limit : Inport  Port=2
  MinMax : DSPBAPrim/MinMax  primtype=minmaxfunc  nInputs=2  nOutputs=1  omode=Inherit via internal rule  otype=sfix(16)  scale=2^-15  rndmethod=Unbiased  factor=1  satmethod=Symmetric  shift_vec=[0 1 2 -1]  value=0  inPortNames=[' '; ' ';]  outPortNames=[' ']  dspbaimage=dspba_prim.jpg  text=disp('min');  style=Optimised  visibilities=8+2^17  functionExpr=min  advOptions=[]  version=20121130
  MinMax1 : DSPBAPrim/MinMax  primtype=minmaxfunc  nInputs=2  nOutputs=1  omode=Inherit via internal rule  otype=sfix(16)  scale=2^-15  rndmethod=Unbiased  factor=1  satmethod=Symmetric  shift_vec=[0 1 2 -1]  value=0  inPortNames=[' '; ' ';]  outPortNames=[' ']  dspbaimage=dspba_prim.jpg  text=disp('min');  style=Optimised  visibilities=8+2^17  functionExpr=max  advOptions=[]  version=20121130
  Sub : DSPBAPrim/Sub  primtype=sub  nInputs=2  nOutputs=1  omode=Inherit via internal rule  otype=sfix(16)  scale=2^-15  rndmethod=Unbiased  factor=1  satmethod=Symmetric  shift_vec=[0 1 2 -1]  value=0  inPortNames=['+'; '-';]  outPortNames=[' ']  dspbaimage=dspba_prim.jpg  text=fprintf('-');  style=Optimised  visibilities=8  floatRounding=faithful  advOptions=[]  version=20130115
  lmax : DSPBAPrim/Const  primtype=const  nInputs=0  nOutputs=1  omode=Specify via dialog  otype=fpDT  scale=1  rndmethod=Unbiased  factor=1  satmethod=Symmetric  shift_vec=[0 1 2 -1]  value=0  inPortNames=['+'; '+';]  outPortNames=[' ']  dspbaimage=dspba_prim.jpg  text=fprintf('%s', num2str(value));  style=Optimised  visibilities=8 + 1024  floatPrecision=float32_m23  version=20120820
  q : Outport
  wires:
  MinMax/1 -> MinMax1/1
  MinMax1/1 -> q/1
  Sub/1 -> MinMax1/2
  a/1 -> MinMax/2
  limit/1 -> Sub/2, MinMax/1
  lmax/1 -> Sub/1

== system foc_blocks/FL_float/FPSaturate2 ==
  a : Inport
  limit : Inport  Port=2
  MinMax : DSPBAPrim/MinMax  primtype=minmaxfunc  nInputs=2  nOutputs=1  omode=Inherit via internal rule  otype=sfix(16)  scale=2^-15  rndmethod=Unbiased  factor=1  satmethod=Symmetric  shift_vec=[0 1 2 -1]  value=0  inPortNames=[' '; ' ';]  outPortNames=[' ']  dspbaimage=dspba_prim.jpg  text=disp('min');  style=Optimised  visibilities=8+2^17  functionExpr=min  advOptions=[]  version=20121130
  MinMax1 : DSPBAPrim/MinMax  primtype=minmaxfunc  nInputs=2  nOutputs=1  omode=Inherit via internal rule  otype=sfix(16)  scale=2^-15  rndmethod=Unbiased  factor=1  satmethod=Symmetric  shift_vec=[0 1 2 -1]  value=0  inPortNames=[' '; ' ';]  outPortNames=[' ']  dspbaimage=dspba_prim.jpg  text=disp('min');  style=Optimised  visibilities=8+2^17  functionExpr=max  advOptions=[]  version=20121130
  Sub : DSPBAPrim/Sub  primtype=sub  nInputs=2  nOutputs=1  omode=Inherit via internal rule  otype=sfix(16)  scale=2^-15  rndmethod=Unbiased  factor=1  satmethod=Symmetric  shift_vec=[0 1 2 -1]  value=0  inPortNames=['+'; '-';]  outPortNames=[' ']  dspbaimage=dspba_prim.jpg  text=fprintf('-');  style=Optimised  visibilities=8  floatRounding=faithful  advOptions=[]  version=20130115
  lmax : DSPBAPrim/Const  primtype=const  nInputs=0  nOutputs=1  omode=Specify via dialog  otype=fpDT  scale=1  rndmethod=Unbiased  factor=1  satmethod=Symmetric  shift_vec=[0 1 2 -1]  value=0  inPortNames=['+'; '+';]  outPortNames=[' ']  dspbaimage=dspba_prim.jpg  text=fprintf('%s', num2str(value));  style=Optimised  visibilities=8 + 1024  floatPrecision=float32_m23  version=20120820
  q : Outport
  wires:
  lmax/1 -> Sub/1
  limit/1 -> MinMax/1, Sub/2
  a/1 -> MinMax/2
  Sub/1 -> MinMax1/2
  MinMax1/1 -> q/1
  MinMax/1 -> MinMax1/1

== system foc_blocks/FL_float/FP_CP1_DSPBA1 ==
  note: Park & Clarke Transform
  I_uw : Inport
  cos_phi_el : Inport  Port=2
  sin_phi_el : Inport  Port=3
  Add : DSPBAPrim/Add  primtype=add  nInputs=evalAionMaskParam(gcb,'value',1)  nOutputs=1  omode=Inherit via internal rule  otype=sfix(16)  scale=2^-15  rndmethod=Unbiased  factor=1  satmethod=Symmetric  shift_vec=[0 1 2 -1]  value=2  inPortNames=[' '; ' ';]  outPortNames=[' ']  dspbaimage=dspba_prim.jpg  text=fprintf('+');  style=Optimised  visibilities=1032  genFPC=off  floatRounding=faithful  advOptions=[]  version=20130821
  Add1 : DSPBAPrim/Add  primtype=add  nInputs=evalAionMaskParam(gcb,'value',1)  nOutputs=1  omode=Inherit via internal rule with word growth  otype=sfix(16)  scale=2^-15  rndmethod=Unbiased  factor=1  satmethod=Symmetric  shift_vec=[0 1 2 -1]  value=2  inPortNames=[' '; ' ';]  outPortNames=[' ']  dspbaimage=dspba_prim.jpg  text=fprintf('+');  style=Optimised  visibilities=1032  genFPC=off  floatRounding=faithful  advOptions=[]  version=20130821
  Altera DSP Builder Advanced : AlteraGenericMotorLibrary/FP_Cur_Ctrl_DSPBA/Altera DSP Builder Advanced  SystemSampleTime=-1  VariantActivationTime=update diagram  Latency=0  AutoFrameSizeCalculation=off
  Demux1 : Demux  Outputs=2
  FPGain : Subsystem  mask{constVal=2}
      mask prompts: constVal "Gain"
      mask Display: color('w');fprintf('FP Gain\n%s', num2str(constVal));port_label('input',1,'a');port_label('output',1,'q');
  FPGain1 : Subsystem  mask{constVal=-1/sqrt(3)}
      mask prompts: constVal "Gain"
      mask Display: color('w');fprintf('FP Gain\n%s', num2str(constVal));port_label('input',1,'a');port_label('output',1,'q');
  Mult{,1..3} (4 alike) : DSPBAPrim/Mult  primtype=mult  nInputs=2  nOutputs=1  omode=Inherit via internal rule  otype=sfix(16)  scale=2^-15  rndmethod=Unbiased  factor=1  satmethod=Symmetric  shift_vec=[0 1 2 -1]  value=0  inPortNames=[' '; ' ';]  outPortNames=[' ']  dspbaimage=dspba_prim.jpg  text=fprintf('X');  style=Optimised  visibilities=8  floatPrecision=float32_m23  floatRounding=faithful  advOptions=[]  version=20130115
  Mux1 : Mux  Inputs=2
  Sub1 : DSPBAPrim/Sub  primtype=sub  nInputs=2  nOutputs=1  omode=Inherit via internal rule  otype=sfix(16)  scale=2^-15  rndmethod=Unbiased  factor=1  satmethod=Symmetric  shift_vec=[0 1 2 -1]  value=0  inPortNames=['+'; '-';]  outPortNames=[' ']  dspbaimage=dspba_prim.jpg  text=fprintf('-');  style=Optimised  visibilities=8  floatRounding=faithful  advOptions=[]  version=20130115
  I_dq : Outport
  wires:
  FPGain/1(Out1) -> Add1/2
  Add1/1 -> FPGain1/1(In1)
  sin_phi_el/1 -> Mult2/1, Mult1/2
  I_uw/1 -> Demux1/1
  Demux1/2 -> FPGain/1(In1)
  Demux1/1 -> Add1/1, Mult2/2, Mult/1
  FPGain1/1(Out1) -> Mult3/1, Mult1/1
  cos_phi_el/1 -> Mult3/2, Mult/2
  Mult/1 -> Add/1
  Mult1/1 -> Add/2
  Mult2/1 -> Sub1/2
  Mult3/1 -> Sub1/1
  Mux1/1 -> I_dq/1
  Add/1 -> Mux1/1
  Sub1/1 -> Mux1/2

== system foc_blocks/FL_float/FP_Inv_Park1 ==
  note: Inverse Park Transform
  I_dq : Inport
  cos_phi_el : Inport  Port=2
  sin_phi_el : Inport  Port=3
  Add : DSPBAPrim/Add  primtype=add  nInputs=evalAionMaskParam(gcb,'value',1)  nOutputs=1  omode=Inherit via internal rule  otype=sfix(16)  scale=2^-15  rndmethod=Unbiased  factor=1  satmethod=Symmetric  shift_vec=[0 1 2 -1]  value=2  inPortNames=[' '; ' ';]  outPortNames=[' ']  dspbaimage=dspba_prim.jpg  text=fprintf('+');  style=Optimised  visibilities=1032  genFPC=off  floatRounding=faithful  advOptions=[]  version=20130821
  Altera DSP Builder Advanced : AlteraGenericMotorLibrary/FP_Cur_Ctrl_DSPBA/Altera DSP Builder Advanced  SystemSampleTime=-1  VariantActivationTime=update diagram  Latency=0  AutoFrameSizeCalculation=off
  Demux1 : Demux  Outputs=2
  Mult{1..4} (4 alike) : DSPBAPrim/Mult  primtype=mult  nInputs=2  nOutputs=1  omode=Inherit via internal rule  otype=sfix(16)  scale=2^-15  rndmethod=Unbiased  factor=1  satmethod=Symmetric  shift_vec=[0 1 2 -1]  value=0  inPortNames=[' '; ' ';]  outPortNames=[' ']  dspbaimage=dspba_prim.jpg  text=fprintf('X');  style=Optimised  visibilities=8  floatPrecision=float32_m23  floatRounding=faithful  advOptions=[]  version=20130115
  Mux2 : Mux  Inputs=2
  Sub1 : DSPBAPrim/Sub  primtype=sub  nInputs=2  nOutputs=1  omode=Inherit via internal rule  otype=sfix(16)  scale=2^-15  rndmethod=Unbiased  factor=1  satmethod=Symmetric  shift_vec=[0 1 2 -1]  value=0  inPortNames=['+'; '-';]  outPortNames=[' ']  dspbaimage=dspba_prim.jpg  text=fprintf('-');  style=Optimised  visibilities=8  floatRounding=faithful  advOptions=[]  version=20130115
  I_alpha_beta : Outport
  wires:
  Add/1 -> Mux2/2
  Sub1/1 -> Mux2/1
  Mux2/1 -> I_alpha_beta/1
  I_dq/1 -> Demux1/1
  sin_phi_el/1 -> Mult3/2, Mult2/2
  Demux1/2 -> Mult3/1, Mult1/1  "I_q"
  cos_phi_el/1 -> Mult4/2, Mult1/2
  Demux1/1 -> Mult4/1, Mult2/1  "I_d"
  Mult3/1 -> Sub1/2
  Mult4/1 -> Sub1/1
  Mult1/1 -> Add/2
  Mult2/1 -> Add/1

== system foc_blocks/FL_float/PI_Ctrl_D_DSPBA ==
  note: Integral Input
  note: Integral Output
  note: Correction Output
  note: Saturate
  note: Saturate
  note: Integral Gain
  note: Proportional Gain
  note: Error Input
  note: Simple Proportional + Integral (PI) Controller
  note: Saturation limit
  PI_in : Inport
  Integral_in : Inport  Port=2
  Kp_in : Inport  Port=3
  Ki_in : Inport  Port=4
  Add1 : DSPBAPrim/Add  primtype=add  nInputs=evalAionMaskParam(gcb,'value',1)  nOutputs=1  omode=Inherit via internal rule  otype=fpDT  scale=1  rndmethod=Unbiased  factor=1  satmethod=Symmetric  shift_vec=[0 1 2 -1]  value=2  inPortNames=[' '; ' ';]  outPortNames=[' ']  dspbaimage=dspba_prim.jpg  text=fprintf('+');  style=Optimised  visibilities=1032  genFPC=off  floatRounding=faithful  advOptions=[]  version=20130821
  Add4 : DSPBAPrim/Add  primtype=add  nInputs=evalAionMaskParam(gcb,'value',1)  nOutputs=1  omode=Inherit via internal rule  otype=fpDT  scale=1  rndmethod=Unbiased  factor=1  satmethod=Symmetric  shift_vec=[0 1 2 -1]  value=2  inPortNames=[' '; ' ';]  outPortNames=[' ']  dspbaimage=dspba_prim.jpg  text=fprintf('+');  style=Optimised  visibilities=1032  genFPC=off  floatRounding=faithful  advOptions=[]  version=20130821
  Altera DSP Builder Advanced : AlteraGenericMotorLibrary/FP_Cur_Ctrl_DSPBA/Altera DSP Builder Advanced  SystemSampleTime=-1  VariantActivationTime=update diagram  Latency=0  AutoFrameSizeCalculation=off
  FPSaturate1 : Subsystem
      mask Display: color('w');fprintf('FP Var Sat\n');port_label('input',1,'a');port_label('input',2,'limit');port_label('output',1,'q');
  FPSaturate2 : Subsystem
      mask Display: color('w');fprintf('FP Var Sat\n');port_label('input',1,'a');port_label('input',2,'limit');port_label('output',1,'q');
  Mult1 : DSPBAPrim/Mult  primtype=mult  nInputs=2  nOutputs=1  omode=Inherit via internal rule  otype=sfix(16)  scale=2^-15  rndmethod=Unbiased  factor=1  satmethod=Symmetric  shift_vec=[0 1 2 -1]  value=0  inPortNames=[' '; ' ';]  outPortNames=[' ']  dspbaimage=dspba_prim.jpg  text=fprintf('X');  style=Optimised  visibilities=8  floatPrecision=float32_m23  floatRounding=faithful  advOptions=[]  version=20130115
  Mult4 : DSPBAPrim/Mult  primtype=mult  nInputs=2  nOutputs=1  omode=Inherit via internal rule  otype=sfix(16)  scale=2^-15  rndmethod=Unbiased  factor=1  satmethod=Symmetric  shift_vec=[0 1 2 -1]  value=0  inPortNames=[' '; ' ';]  outPortNames=[' ']  dspbaimage=dspba_prim.jpg  text=fprintf('X');  style=Optimised  visibilities=8  floatPrecision=float32_m23  floatRounding=faithful  advOptions=[]  version=20130115
  Saturation : DSPBAPrim/Const  primtype=const  nInputs=0  nOutputs=1  omode=Specify via dialog  otype=fpDT  scale=1  rndmethod=Unbiased  factor=1  satmethod=Symmetric  shift_vec=[0 1 2 -1]  value=0.95*2^(constwordlengthIn-constfractionlengthIn-1)  inPortNames=['+'; '+';]  outPortNames=[' ']  dspbaimage=dspba_prim.jpg  text=fprintf('%s', num2str(value));  style=Optimised  visibilities=8 + 1024  floatPrecision=float32_m23  version=20120820
  PI_out : Outport
  I_out : Outport  Port=2
  wires:
  Ki_in/1 -> Mult1/2
  Mult1/1 -> Add4/1
  Kp_in/1 -> Mult4/2
  Integral_in/1 -> Add4/2
  Add4/1 -> FPSaturate2/1(a)
  FPSaturate2/1(q) -> I_out/1, Add1/2
  Mult4/1 -> Add1/1
  PI_in/1 -> Mult1/1, Mult4/1
  Add1/1 -> FPSaturate1/1(a)
  FPSaturate1/1(q) -> PI_out/1
  Saturation/1 -> FPSaturate1/2(limit), FPSaturate2/2(limit)

== system foc_blocks/FL_float/PI_Ctrl_Q_DSPBA ==
  note: Simple Proportional + Integral (PI) Controller
  note: Error Input
  note: Proportional Gain
  note: Integral Gain
  note: Saturate
  note: Saturate
  note: Correction Output
  note: Integral Output
  note: Integral Input
  note: Saturation limit
  PI_in : Inport
  Integral_in : Inport  Port=2
  Kp_in : Inport  Port=3
  Ki_in : Inport  Port=4
  Add1 : DSPBAPrim/Add  primtype=add  nInputs=evalAionMaskParam(gcb,'value',1)  nOutputs=1  omode=Inherit via internal rule  otype=fpDT  scale=1  rndmethod=Unbiased  factor=1  satmethod=Symmetric  shift_vec=[0 1 2 -1]  value=2  inPortNames=[' '; ' ';]  outPortNames=[' ']  dspbaimage=dspba_prim.jpg  text=fprintf('+');  style=Optimised  visibilities=1032  genFPC=off  floatRounding=faithful  advOptions=[]  version=20130821
  Add4 : DSPBAPrim/Add  primtype=add  nInputs=evalAionMaskParam(gcb,'value',1)  nOutputs=1  omode=Inherit via internal rule  otype=fpDT  scale=1  rndmethod=Unbiased  factor=1  satmethod=Symmetric  shift_vec=[0 1 2 -1]  value=2  inPortNames=[' '; ' ';]  outPortNames=[' ']  dspbaimage=dspba_prim.jpg  text=fprintf('+');  style=Optimised  visibilities=1032  genFPC=off  floatRounding=faithful  advOptions=[]  version=20130821
  Altera DSP Builder Advanced : AlteraGenericMotorLibrary/FP_Cur_Ctrl_DSPBA/Altera DSP Builder Advanced  SystemSampleTime=-1  VariantActivationTime=update diagram  Latency=0  AutoFrameSizeCalculation=off
  FPSaturate1 : Subsystem
      mask Display: color('w');fprintf('FP Var Sat\n');port_label('input',1,'a');port_label('input',2,'limit');port_label('output',1,'q');
  FPSaturate2 : Subsystem
      mask Display: color('w');fprintf('FP Var Sat\n');port_label('input',1,'a');port_label('input',2,'limit');port_label('output',1,'q');
  Mult1 : DSPBAPrim/Mult  primtype=mult  nInputs=2  nOutputs=1  omode=Inherit via internal rule  otype=sfix(16)  scale=2^-15  rndmethod=Unbiased  factor=1  satmethod=Symmetric  shift_vec=[0 1 2 -1]  value=0  inPortNames=[' '; ' ';]  outPortNames=[' ']  dspbaimage=dspba_prim.jpg  text=fprintf('X');  style=Optimised  visibilities=8  floatPrecision=float32_m23  floatRounding=faithful  advOptions=[]  version=20130115
  Mult4 : DSPBAPrim/Mult  primtype=mult  nInputs=2  nOutputs=1  omode=Inherit via internal rule  otype=sfix(16)  scale=2^-15  rndmethod=Unbiased  factor=1  satmethod=Symmetric  shift_vec=[0 1 2 -1]  value=0  inPortNames=[' '; ' ';]  outPortNames=[' ']  dspbaimage=dspba_prim.jpg  text=fprintf('X');  style=Optimised  visibilities=8  floatPrecision=float32_m23  floatRounding=faithful  advOptions=[]  version=20130115
  Saturation : DSPBAPrim/Const  primtype=const  nInputs=0  nOutputs=1  omode=Specify via dialog  otype=fpDT  scale=1  rndmethod=Unbiased  factor=1  satmethod=Symmetric  shift_vec=[0 1 2 -1]  value=0.95*2^(constwordlengthIn-constfractionlengthIn-1)  inPortNames=['+'; '+';]  outPortNames=[' ']  dspbaimage=dspba_prim.jpg  text=fprintf('%s', num2str(value));  style=Optimised  visibilities=8 + 1024  floatPrecision=float32_m23  version=20120820
  PI_out : Outport
  I_out : Outport  Port=2
  wires:
  FPSaturate1/1(q) -> PI_out/1
  Add1/1 -> FPSaturate1/1(a)
  PI_in/1 -> Mult4/1, Mult1/1
  Mult4/1 -> Add1/1
  FPSaturate2/1(q) -> Add1/2, I_out/1
  Add4/1 -> FPSaturate2/1(a)
  Integral_in/1 -> Add4/2
  Kp_in/1 -> Mult4/2
  Mult1/1 -> Add4/1
  Ki_in/1 -> Mult1/2
  Saturation/1 -> FPSaturate1/2(limit), FPSaturate2/2(limit)

== system foc_blocks/FL_float_filt/FPSaturate1 ==
  a : Inport
  limit : Inport  Port=2
  MinMax : DSPBAPrim/MinMax  primtype=minmaxfunc  nInputs=2  nOutputs=1  omode=Inherit via internal rule  otype=sfix(16)  scale=2^-15  rndmethod=Unbiased  factor=1  satmethod=Symmetric  shift_vec=[0 1 2 -1]  value=0  inPortNames=[' '; ' ';]  outPortNames=[' ']  dspbaimage=dspba_prim.jpg  text=disp('min');  style=Optimised  visibilities=8+2^17  functionExpr=min  advOptions=[]  version=20121130
  MinMax1 : DSPBAPrim/MinMax  primtype=minmaxfunc  nInputs=2  nOutputs=1  omode=Inherit via internal rule  otype=sfix(16)  scale=2^-15  rndmethod=Unbiased  factor=1  satmethod=Symmetric  shift_vec=[0 1 2 -1]  value=0  inPortNames=[' '; ' ';]  outPortNames=[' ']  dspbaimage=dspba_prim.jpg  text=disp('min');  style=Optimised  visibilities=8+2^17  functionExpr=max  advOptions=[]  version=20121130
  Sub : DSPBAPrim/Sub  primtype=sub  nInputs=2  nOutputs=1  omode=Inherit via internal rule  otype=sfix(16)  scale=2^-15  rndmethod=Unbiased  factor=1  satmethod=Symmetric  shift_vec=[0 1 2 -1]  value=0  inPortNames=['+'; '-';]  outPortNames=[' ']  dspbaimage=dspba_prim.jpg  text=fprintf('-');  style=Optimised  visibilities=8  floatRounding=faithful  advOptions=[]  version=20130115
  lmax : DSPBAPrim/Const  primtype=const  nInputs=0  nOutputs=1  omode=Specify via dialog  otype=fpDT  scale=1  rndmethod=Unbiased  factor=1  satmethod=Symmetric  shift_vec=[0 1 2 -1]  value=0  inPortNames=['+'; '+';]  outPortNames=[' ']  dspbaimage=dspba_prim.jpg  text=fprintf('%s', num2str(value));  style=Optimised  visibilities=8 + 1024  floatPrecision=float32_m23  version=20120820
  q : Outport
  wires:
  lmax/1 -> Sub/1
  limit/1 -> MinMax/1, Sub/2
  a/1 -> MinMax/2
  Sub/1 -> MinMax1/2
  MinMax1/1 -> q/1
  MinMax/1 -> MinMax1/1

== system foc_blocks/FL_float_filt/FPSaturate2 ==
  a : Inport
  limit : Inport  Port=2
  MinMax : DSPBAPrim/MinMax  primtype=minmaxfunc  nInputs=2  nOutputs=1  omode=Inherit via internal rule  otype=sfix(16)  scale=2^-15  rndmethod=Unbiased  factor=1  satmethod=Symmetric  shift_vec=[0 1 2 -1]  value=0  inPortNames=[' '; ' ';]  outPortNames=[' ']  dspbaimage=dspba_prim.jpg  text=disp('min');  style=Optimised  visibilities=8+2^17  functionExpr=min  advOptions=[]  version=20121130
  MinMax1 : DSPBAPrim/MinMax  primtype=minmaxfunc  nInputs=2  nOutputs=1  omode=Inherit via internal rule  otype=sfix(16)  scale=2^-15  rndmethod=Unbiased  factor=1  satmethod=Symmetric  shift_vec=[0 1 2 -1]  value=0  inPortNames=[' '; ' ';]  outPortNames=[' ']  dspbaimage=dspba_prim.jpg  text=disp('min');  style=Optimised  visibilities=8+2^17  functionExpr=max  advOptions=[]  version=20121130
  Sub : DSPBAPrim/Sub  primtype=sub  nInputs=2  nOutputs=1  omode=Inherit via internal rule  otype=sfix(16)  scale=2^-15  rndmethod=Unbiased  factor=1  satmethod=Symmetric  shift_vec=[0 1 2 -1]  value=0  inPortNames=['+'; '-';]  outPortNames=[' ']  dspbaimage=dspba_prim.jpg  text=fprintf('-');  style=Optimised  visibilities=8  floatRounding=faithful  advOptions=[]  version=20130115
  lmax : DSPBAPrim/Const  primtype=const  nInputs=0  nOutputs=1  omode=Specify via dialog  otype=fpDT  scale=1  rndmethod=Unbiased  factor=1  satmethod=Symmetric  shift_vec=[0 1 2 -1]  value=0  inPortNames=['+'; '+';]  outPortNames=[' ']  dspbaimage=dspba_prim.jpg  text=fprintf('%s', num2str(value));  style=Optimised  visibilities=8 + 1024  floatPrecision=float32_m23  version=20120820
  q : Outport
  wires:
  MinMax/1 -> MinMax1/1
  MinMax1/1 -> q/1
  Sub/1 -> MinMax1/2
  a/1 -> MinMax/2
  limit/1 -> Sub/2, MinMax/1
  lmax/1 -> Sub/1
